simulink model "dcmotor"  (R2021b)
settings: Solver=FixedStepAuto  StartTime=0.0  StopTime=2.0  FixedStep=0.001  RelTol=1e-3
settings Model: Creator=ПК  LastModifiedBy=ПК

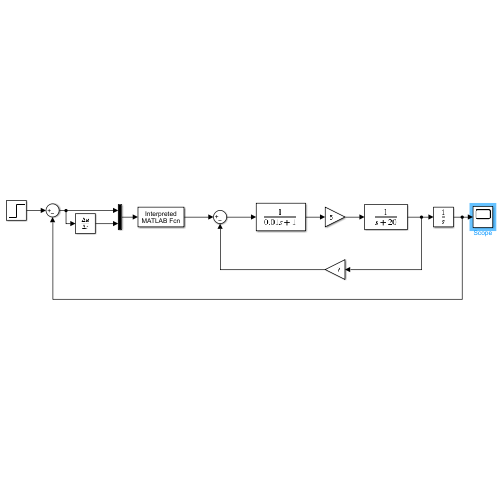
[thumbnail: Simulink's stored preview of the top-level diagram]
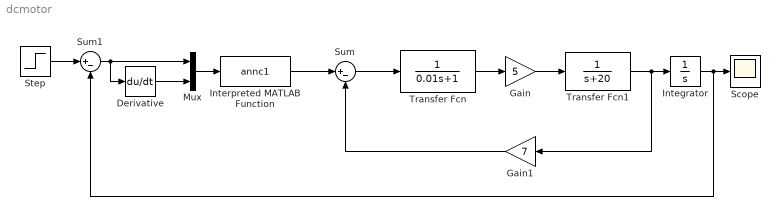
== system dcmotor ==
  Derivative : Derivative
  Gain : Gain  Gain=5
  Gain1 : Gain  Gain=7
  Integrator : Integrator
  Interpreted MATLAB Function : MATLABFcn  MATLABFcn=annc1  OutputDimensions=1
  Mux : Mux  Inputs=2
  Scope : Scope
  Step : Step  Time=0.4  SampleTime=0
  Sum : Sum  Inputs=|+-
  Sum1 : Sum  Inputs=|+-
  Transfer Fcn : TransferFcn  Denominator=[0.01 1]
  Transfer Fcn1 : TransferFcn  Denominator=[1 20]
  wires:
  Transfer Fcn/1 -> Gain/1
  Gain/1 -> Transfer Fcn1/1
  Transfer Fcn1/1 -> Gain1/1, Integrator/1
  Sum/1 -> Transfer Fcn/1
  Gain1/1 -> Sum/2
  Interpreted MATLAB Function/1 -> Sum/1
  Mux/1 -> Interpreted MATLAB Function/1
  Derivative/1 -> Mux/2
  Sum1/1 -> Derivative/1, Mux/1
  Step/1 -> Sum1/1
  Integrator/1 -> Sum1/2, Scope/1
